simulink model "Modele_LQR_6DOF"  (R2025b)
settings: Solver=VariableStepAuto  StartTime=0.0  StopTime=300  FixedStep=0.033333  RelTol=1e-3
values from neighbouring files (symbols this model uses):
  B = -234.459    [AUV_Params.sldd]    (also in block_compute_K.m = [ [                                          0,             )
  Fx1 = -14.142    [AUV_Params.sldd]
  Fx2 = -14.142    [AUV_Params.sldd]
  Fx3 = 0.0    [AUV_Params.sldd]
  Fx4 = 0.0    [AUV_Params.sldd]
  Fx5 = 0.0    [AUV_Params.sldd]
  Fx6 = 0.0    [AUV_Params.sldd]
  Fx7 = 14.142    [AUV_Params.sldd]
  Fx8 = 14.142    [AUV_Params.sldd]
  Fy1 = 14.142    [AUV_Params.sldd]
  Fy2 = -14.142    [AUV_Params.sldd]
  Fy3 = 0.0    [AUV_Params.sldd]
  Fy4 = 0.0    [AUV_Params.sldd]
  Fy5 = 0.0    [AUV_Params.sldd]
  Fy6 = 0.0    [AUV_Params.sldd]
  Fy7 = 14.142    [AUV_Params.sldd]
  Fy8 = -14.142    [AUV_Params.sldd]
  Fz1 = 0.0    [AUV_Params.sldd]
  Fz2 = 0.0    [AUV_Params.sldd]
  Fz3 = -20.0    [AUV_Params.sldd]
  Fz4 = -20.0    [AUV_Params.sldd]
  Fz5 = -20.0    [AUV_Params.sldd]
  Fz6 = -20.0    [AUV_Params.sldd]
  Fz7 = 0.0    [AUV_Params.sldd]
  Fz8 = 0.0    [AUV_Params.sldd]
  I_x = 0.578    [AUV_Params.sldd]
  I_y = 0.645    [AUV_Params.sldd]
  I_z = 0.9366    [AUV_Params.sldd]
  lx1 = 0.0194    [AUV_Params.sldd]
  lx2 = 0.0194    [AUV_Params.sldd]
  lx3 = -0.0317    [AUV_Params.sldd]
  lx4 = -0.0317    [AUV_Params.sldd]
  lx5 = 0.0317    [AUV_Params.sldd]
  lx6 = 0.0317    [AUV_Params.sldd]
  lx7 = -0.0194    [AUV_Params.sldd]
  lx8 = -0.0194    [AUV_Params.sldd]
  ly1 = 0.0381    [AUV_Params.sldd]
  ly2 = -0.0381    [AUV_Params.sldd]
  ly3 = 0.0049    [AUV_Params.sldd]
  ly4 = -0.0049    [AUV_Params.sldd]
  ly5 = 0.0049    [AUV_Params.sldd]
  ly6 = -0.0049    [AUV_Params.sldd]
  ly7 = 0.0381    [AUV_Params.sldd]
  ly8 = -0.0381    [AUV_Params.sldd]
  lz1 = 0.0575    [AUV_Params.sldd]
  lz2 = 0.0575    [AUV_Params.sldd]
  lz3 = 0.0366    [AUV_Params.sldd]
  lz4 = 0.0366    [AUV_Params.sldd]
  lz5 = 0.0366    [AUV_Params.sldd]
  lz6 = 0.0366    [AUV_Params.sldd]
  lz7 = 0.0575    [AUV_Params.sldd]
  lz8 = 0.0575    [AUV_Params.sldd]
  m = 23.9    [AUV_Params.sldd]
  W = 234.459    [AUV_Params.sldd]
  x_rb = 0.0    [AUV_Params.sldd]
  x_rg = 0.0    [AUV_Params.sldd]
  y_rb = 0.0    [AUV_Params.sldd]
  y_rg = 0.0    [AUV_Params.sldd]
  z_rb = 0.0    [AUV_Params.sldd]
  z_rg = 0.0    [AUV_Params.sldd]
undefined symbols (not defined in the file or in its folder): A_num, Q_envoyer, sigbuilder_block, SIZE_TRAJ, T_TRAJ, TRAJECTOIRE, YAW_MODE
libraries: simulink x12, sharedtransform x1, dspinverses x1, SignalEditorBlockLib x1
(part 2 of 4)

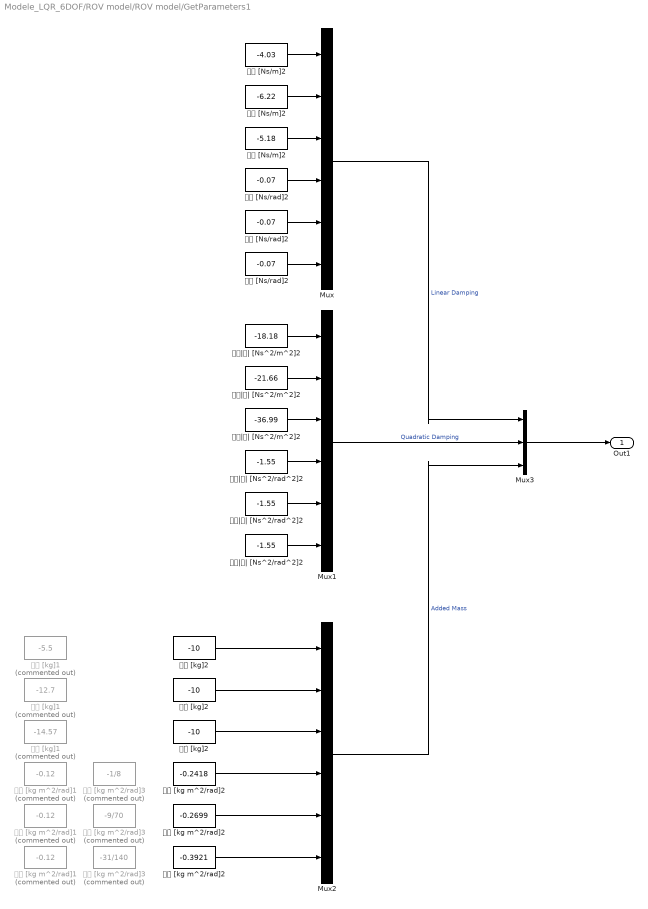
== system Modele_LQR_6DOF/ROV model/ROV model/GetParameters1 ==
  Mux : Mux  Inputs=6
  Mux1 : Mux  Inputs=6
  Mux2 : Mux  Inputs=6
  Mux3 : Mux  Inputs=3
  𝐾𝑝 [Ns/rad]2 : Constant  Value=-0.07
  𝐾𝑝|𝑝| [Ns^2/rad^2]2 : Constant  Value=-1.55
  𝐾𝑝̇ [kg m^2/rad]1 : Constant  Commented=on  Value=-0.12
  𝐾𝑝̇ [kg m^2/rad]2 : Constant  Value=-0.2418
  𝐾𝑝̇ [kg m^2/rad]3 : Constant  Commented=on  Value=-1/8
  𝑀𝑞 [Ns/rad]2 : Constant  Value=-0.07
  𝑀𝑞|𝑞| [Ns^2/rad^2]2 : Constant  Value=-1.55
  𝑀𝑞̇ [kg m^2/rad]1 : Constant  Commented=on  Value=-0.12
  𝑀𝑞̇ [kg m^2/rad]2 : Constant  Value=-0.2699
  𝑀𝑞̇ [kg m^2/rad]3 : Constant  Commented=on  Value=-9/70
  𝑁𝑟 [Ns/rad]2 : Constant  Value=-0.07
  𝑁𝑟|𝑟| [Ns^2/rad^2]2 : Constant  Value=-1.55
  𝑁𝑟̇ [kg m^2/rad]1 : Constant  Commented=on  Value=-0.12
  𝑁𝑟̇ [kg m^2/rad]2 : Constant  Value=-0.3921
  𝑁𝑟̇ [kg m^2/rad]3 : Constant  Commented=on  Value=-31/140
  𝑋𝑢 [Ns/m]2 : Constant  Value=-4.03
  𝑋𝑢|𝑢| [Ns^2/m^2]2 : Constant  Value=-18.18
  𝑋𝑢̇ [kg]1 : Constant  Commented=on  Value=-5.5
  𝑋𝑢̇ [kg]2 : Constant  Value=-10
  𝑌𝑣 [Ns/m]2 : Constant  Value=-6.22
  𝑌𝑣|𝑣| [Ns^2/m^2]2 : Constant  Value=-21.66
  𝑌𝑣̇ [kg]1 : Constant  Commented=on  Value=-12.7
  𝑌𝑣̇ [kg]2 : Constant  Value=-10
  𝑍𝑤 [Ns/m]2 : Constant  Value=-5.18
  𝑍𝑤|𝑤| [Ns^2/m^2]2 : Constant  Value=-36.99
  𝑍𝑤̇ [kg]1 : Constant  Commented=on  Value=-14.57
  𝑍𝑤̇ [kg]2 : Constant  Value=-10
  Out1 : Outport  VectorParamsAs1DForOutWhenUnconnected=off
  wires:
  𝑁𝑟 [Ns/rad]2/1 -> Mux/6
  Mux/1 -> Mux3/1  "Linear Damping"
  𝐾𝑝 [Ns/rad]2/1 -> Mux/4
  𝑀𝑞 [Ns/rad]2/1 -> Mux/5
  𝑍𝑤 [Ns/m]2/1 -> Mux/3
  𝑌𝑣 [Ns/m]2/1 -> Mux/2
  𝑋𝑢 [Ns/m]2/1 -> Mux/1
  𝑌𝑣|𝑣| [Ns^2/m^2]2/1 -> Mux1/2
  𝑍𝑤|𝑤| [Ns^2/m^2]2/1 -> Mux1/3
  𝑋𝑢|𝑢| [Ns^2/m^2]2/1 -> Mux1/1
  Mux1/1 -> Mux3/2  "Quadratic Damping"
  𝑀𝑞|𝑞| [Ns^2/rad^2]2/1 -> Mux1/5
  𝑁𝑟|𝑟| [Ns^2/rad^2]2/1 -> Mux1/6
  𝐾𝑝|𝑝| [Ns^2/rad^2]2/1 -> Mux1/4
  Mux2/1 -> Mux3/3  "Added Mass"
  Mux3/1 -> Out1/1
  𝑋𝑢̇ [kg]2/1 -> Mux2/1
  𝑌𝑣̇ [kg]2/1 -> Mux2/2
  𝑍𝑤̇ [kg]2/1 -> Mux2/3
  𝐾𝑝̇ [kg m^2/rad]2/1 -> Mux2/4
  𝑀𝑞̇ [kg m^2/rad]2/1 -> Mux2/5
  𝑁𝑟̇ [kg m^2/rad]2/1 -> Mux2/6

== matlab function Modele_LQR_6DOF/Controller/Gestionnaire des Vitesses/MATLAB Function1 ==
  data: xstate input; u output; xtarget input
function u = fcn(xstate,xtarget)

precition = 0.01;
% precition = 0.01; % originalt

if(xstate < xtarget - precition)
    u = 1; % original (1)

elseif(xstate > xtarget + precition)
    u = -1; % original (1)
    
else
    u = 0;
end
end

== matlab function Modele_LQR_6DOF/Controller/Gestionnaire des Vitesses/MATLAB Function ==
  data: xstate input; u output; xtarget input
function u = fcn(xstate,xtarget)

precition = 0.01;
% precition = 0.01; % original

if(xstate < xtarget - precition)
    u = 1; % original (1)

elseif(xstate > xtarget + precition)
    u = -1; % original (1)
    
else
    u = 0;
end
end

== matlab function Modele_LQR_6DOF/ROV model/ROV model/Kinetics1 ==
  data: u input size=1; u_dot output; v input size=1; w input size=1; p input size=1; q input size=1; r input size=1; phi input; theta input; psi input; tau input; v_dot output; w_dot output; p_dot output; q_dot output; r_dot output; u_dot_temp input; v_dot_temp input; w_dot_temp input; p_dot_temp input; q_dot_temp input; r_dot_temp input; disturbance input; EstimatedParams input; B parameter; Fx1 input; Fx2 input; Fx3 input; Fx4 input; Fx5 input; Fx6 input; Fx7 input; Fx8 input; Fy1 input; Fy2 input; Fy3 input; Fy4 input; Fy5 input; Fy6 input; Fy7 input; Fy8 input; Fz1 input; Fz2 input; Fz3 input; Fz4 input; Fz5 input; Fz6 input; Fz7 input; Fz8 input; I_x input; I_y input; I_z input; lx1 input; lx2 input; lx3 input; lx4 input; lx5 input; lx6 input; lx7 input; lx8 input; ly1 input; ly2 input; ly3 input; ly4 input; ly5 input; ly6 input; ly7 input; ly8 input; lz1 input; lz2 input; lz3 input; lz4 input; lz5 input; lz6 input; lz7 input; lz8 input; m parameter; W parameter; x_rb parameter; x_rg parameter; y_rb parameter; y_rg parameter; z_rb parameter; z_rg parameter
function [u_dot,v_dot,w_dot,p_dot,q_dot,r_dot] = Kinetics1(u,v,w,p,q,r,phi,theta,psi,tau,u_dot_temp,v_dot_temp,w_dot_temp,p_dot_temp,q_dot_temp,r_dot_temp, disturbance,EstimatedParams, B, Fx1, Fx2, Fx3, Fx4, Fx5, Fx6, Fx7, Fx8, Fy1, Fy2, Fy3, Fy4, Fy5, Fy6, Fy7, Fy8, Fz1, Fz2, Fz3, Fz4, Fz5, Fz6, Fz7, Fz8, I_x, I_y, I_z, lx1, lx2, lx3, lx4, lx5, lx6, lx7, lx8, ly1, ly2, ly3, ly4, ly5, ly6, ly7, ly8, lz1, lz2, lz3, lz4, lz5, lz6, lz7, lz8, m, W, x_rb, x_rg, y_rb, y_rg, z_rb, z_rg)
% LIVRE HMCH PAGE 58
%extract forces from thrusters
f1=tau(1);
f2=tau(2);
f3=tau(3);
f4=tau(4);
f5=tau(5);
f6=tau(6);
f7=tau(7);
f8=tau(8);
x_rb = 0; x_rg = 0; y_rb = 0; y_rg = 0; z_rb = 0; z_rg = 0;
  displaced_water_volume = 0.03; % 0.03
  water_density = 1000.0;
  radius = 0.26;
  m = 23.9;
  g = 9.81;
  W = m * g;
  % B = water_density*displaced_water_volume*g;
  B = W;
%extract estimated parameters
X_u = EstimatedParams(1);
Y_v = EstimatedParams(2);
Z_w = EstimatedParams(3);
K_p = EstimatedParams(4); 
M_q = EstimatedParams(5);
N_r = EstimatedParams(6);
X_uu = EstimatedParams(7);
Y_vv = EstimatedParams(8);
Z_ww = EstimatedParams(9);
K_pp = EstimatedParams(10); 
M_qq = EstimatedParams(11); 
N_rr = EstimatedParams(12);
X_u_dot = EstimatedParams(13);
Y_v_dot = EstimatedParams(14);
Z_w_dot = EstimatedParams(15);
K_p_dot = EstimatedParams(16);
M_q_dot = EstimatedParams(17); 
N_r_dot = EstimatedParams(18); 
%extract forces from disturbance
u_c = disturbance(1);
v_c = disturbance(2);
w_c = disturbance(3);
p_c = disturbance(4);
q_c = disturbance(5);
r_c = disturbance(6);
%Full Equations without disturbance with zg = 0.02
% u_dot = -((0.7071*f1) + (0.7071*f2) - (0.7071*f3) - (0.7071*f4)- (0.230*q_dot_temp) + 2*sin(theta) + u*(X_u + X_uu*abs(u)) - (0.230*p*r) - (11.50*q*w) + (11.50*r*v) - Y_v_dot*r*v + Z_w_dot*q*w)/(X_u_dot - 11.50);
% v_dot = ((0.7071*f1) - (0.7071*f2) + (0.7071*f3) - (0.7071*f4) - (0.230*p_dot_temp) + 2*cos(theta)*sin(phi) - v*(Y_v + Y_vv*abs(v)) + (11.50*q*r) - (11.50*p*w) + (11.50*r*u) - X_u_dot*r*u + Z_w_dot*p*w)/(Y_v_dot - 11.50);
% w_dot = -(f6 - f5 + f7 - f8 - 2*cos(phi)*cos(theta) + w*(Z_w + Z_ww*abs(w)) + q*((23*q)/100 - X_u_dot*u) + p*((23*p)/100 + Y_v_dot*v) - (11.50*p*v) + (11.50*q*u))/(Z_w_dot - 11.50);
% p_dot = -(25*((0.0601*f1) - (0.0601*f2) + (0.0601*f3) - (0.0601*f4) - (109*f5)/500 - (109*f6)/500 + (0.2180*f7) + (0.2180*f8) + (0.230*v_dot_temp) + K_p*p - (2.2560*cos(theta)*sin(phi)) - (0.230*p*w) + (0.230*r*u) - M_q_dot*q*r + N_r_dot*q*r - Y_v_dot*v*w + Z_w_dot*v*w + K_pp*p*abs(p)))/(25*K_p_dot - 4);
% q_dot =-(25*((0.0601*f1) + (0.0601*f2) - (0.0601*f3) - (0.0601*f4)+ (0.120*f5) - (0.120*f6) + (0.120*f7) - (0.120*f8) - (0.230*u_dot_temp) - (2.2560*sin(theta)) + M_q*q - (0.230*q*w) + (0.230*r*v) + K_p_dot*p*r - N_r_dot*p*r + X_u_dot*u*w - Z_w_dot*u*w + M_qq*q*abs(q)))/(25*M_q_dot - 4);
% r_dot = -(25*((0.1888*f2) - (0.1888*f1) + (0.1888*f3) - (0.1888*f4) + N_r*r - K_p_dot*p*q + M_q_dot*p*q - X_u_dot*u*v + Y_v_dot*u*v + N_rr*r*abs(r)))/(25*N_r_dot - 4);

%Full Equations without disturbance with zg = 0.02 + utilisation de la fontion vpa
% u_dot = -(1.0*(0.7071*f1 + 0.7071*f2 - 0.7071*f3 - 0.7071*f4 - 0.23*q_dot_temp + 2.0*sin(theta) + (X_u + X_uu*abs(u - 1.0*u_c))*(u - 1.0*u_c) - 1.0*(11.5*q - 11.5*q_c)*(w - 1.0*w_c) + (11.5*r - 11.5*r_c)*(v - 1.0*v_c) - 1.0*(p - 1.0*p_c)*(0.23*r - 0.23*r_c) + (X_u_dot - 11.5)*(q*w_c - 1.0*r*v_c) - 1.0*Y_v_dot*(r - 1.0*r_c)*(v - 1.0*v_c) + Z_w_dot*(q - 1.0*q_c)*(w - 1.0*w_c)))/(X_u_dot - 11.5);
% v_dot = (0.7071*f1 - 0.7071*f2 + 0.7071*f3 - 0.7071*f4 - 0.23*p_dot_temp - 1.0*(11.5*p - 11.5*p_c)*(w - 1.0*w_c) + (11.5*r - 11.5*r_c)*(u - 1.0*u_c) - 1.0*(Y_v + Y_vv*abs(v - 1.0*v_c))*(v - 1.0*v_c) + 2.0*cos(theta)*sin(phi) + (q - 1.0*q_c)*(0.23*r - 0.23*r_c) + (Y_v_dot - 11.5)*(p*w_c - 1.0*r*u_c) - 1.0*X_u_dot*(r - 1.0*r_c)*(u - 1.0*u_c) + Z_w_dot*(p - 1.0*p_c)*(w - 1.0*w_c))/(Y_v_dot - 11.5);
% w_dot =-(1.0*(f6 - 1.0*f5 + f7 - 1.0*f8 - 1.0*(11.5*p - 11.5*p_c)*(v - 1.0*v_c) + (11.5*q - 11.5*q_c)*(u - 1.0*u_c) - 2.0*cos(phi)*cos(theta) + (Z_w + Z_ww*abs(w - 1.0*w_c))*(w - 1.0*w_c) + (Z_w_dot - 11.5)*(p*v_c - 1.0*q*u_c) + (p - 1.0*p_c)*(0.23*p - 0.23*p_c + Y_v_dot*(v - 1.0*v_c)) - 1.0*(q - 1.0*q_c)*(0.23*q_c - 0.23*q + X_u_dot*(u - 1.0*u_c))))/(Z_w_dot - 11.5);
% p_dot =-(1.0*(0.0601035*f1 - 0.0601035*f2 + 0.0601035*f3 - 0.0601035*f4 - 0.218*f5 - 0.218*f6 + 0.218*f7 + 0.218*f8 + 0.23*v_dot - 2.256*cos(theta)*sin(phi) + (u - 1.0*u_c)*(0.23*r - 0.23*r_c) - 0.23*p*w_c + 0.23*r*u_c - 1.0*(r - 1.0*r_c)*(0.16*q_c - 0.16*q + M_q_dot*(q - 1.0*q_c)) + (q - 1.0*q_c)*(0.16*r_c - 0.16*r + N_r_dot*(r - 1.0*r_c)) + (K_p + K_pp*abs(p - 1.0*p_c))*(p - 1.0*p_c) - 1.0*(w - 1.0*w_c)*(0.23*p - 0.23*p_c + Y_v_dot*(v - 1.0*v_c)) + Z_w_dot*(v - 1.0*v_c)*(w - 1.0*w_c)))/(K_p_dot - 0.16);
% q_dot =-(1.0*(0.0601035*f1 + 0.0601035*f2 - 0.0601035*f3 - 0.0601035*f4 + 0.12*f5 - 0.12*f6 + 0.12*f7 - 0.12*f8 - 0.23*u_dot - 2.256*sin(theta) + (v - 1.0*v_c)*(0.23*r - 0.23*r_c) - 0.23*q*w_c + 0.23*r*v_c + (r - 1.0*r_c)*(0.16*p_c - 0.16*p + K_p_dot*(p - 1.0*p_c)) - 1.0*(p - 1.0*p_c)*(0.16*r_c - 0.16*r + N_r_dot*(r - 1.0*r_c)) + (w - 1.0*w_c)*(0.23*q_c - 0.23*q + X_u_dot*(u - 1.0*u_c)) + (M_q + M_qq*abs(q - 1.0*q_c))*(q - 1.0*q_c) - 1.0*Z_w_dot*(u - 1.0*u_c)*(w - 1.0*w_c)))/(M_q_dot - 0.16);
% r_dot = -(1.0*(0.1887957*f2 - 0.1887957*f1 + 0.1887957*f3 - 0.1887957*f4 - 1.0*(q - 1.0*q_c)*(0.16*p_c - 0.16*p + K_p_dot*(p - 1.0*p_c)) + (p - 1.0*p_c)*(0.16*q_c - 0.16*q + M_q_dot*(q - 1.0*q_c)) + (N_r + N_rr*abs(r - 1.0*r_c))*(r - 1.0*r_c) - 1.0*X_u_dot*(u - 1.0*u_c)*(v - 1.0*v_c) + Y_v_dot*(u - 1.0*u_c)*(v - 1.0*v_c)))/(N_r_dot - 0.16);

% u_dot = -(1.0*((X_u + X_uu*abs(u - 1.0*u_c))*(u - 1.0*u_c) + sin(theta)*(B - 9.81*m) + Fx1*f1 + Fx2*f2 + Fx3*f3 + Fx4*f4 + Fx5*f5 + Fx6*f6 + Fx7*f7 + Fx8*f8 + (q*w_c - 1.0*r*v_c)*(X_u_dot - 1.0*m) + (Z_w_dot*(w - 1.0*w_c) + m*x_rg*(q - 1.0*q_c))*(q - 1.0*q_c) - 1.0*(Y_v_dot*(v - 1.0*v_c) - 1.0*m*x_rg*(r - 1.0*r_c))*(r - 1.0*r_c) - 1.0*(m*y_rg*(q - 1.0*q_c) + m*z_rg*(r - 1.0*r_c))*(p - 1.0*p_c) - 1.0*m*(q - 1.0*q_c)*(w - 1.0*w_c) + m*(r - 1.0*r_c)*(v - 1.0*v_c) - 1.0*m*q_dot_temp*z_rg + m*r_dot_temp*y_rg))/(X_u_dot - 1.0*m);
%  
%  
% v_dot = -(1.0*((Y_v + Y_vv*abs(v - 1.0*v_c))*(v - 1.0*v_c) + Fy1*f1 + Fy2*f2 + Fy3*f3 + Fy4*f4 + Fy5*f5 + Fy6*f6 + Fy7*f7 + Fy8*f8 - 1.0*(p*w_c - 1.0*r*u_c)*(Y_v_dot - 1.0*m) + (X_u_dot*(u - 1.0*u_c) + m*y_rg*(r - 1.0*r_c))*(r - 1.0*r_c) - 1.0*(Z_w_dot*(w - 1.0*w_c) - 1.0*m*y_rg*(p - 1.0*p_c))*(p - 1.0*p_c) - 1.0*(m*x_rg*(p - 1.0*p_c) + m*z_rg*(r - 1.0*r_c))*(q - 1.0*q_c) + m*(p - 1.0*p_c)*(w - 1.0*w_c) - 1.0*m*(r - 1.0*r_c)*(u - 1.0*u_c) + m*p_dot_temp*z_rg - 1.0*m*r_dot_temp*x_rg - 1.0*cos(theta)*sin(phi)*(B - 9.81*m)))/(Y_v_dot - 1.0*m);
%  
%  
% w_dot = -(1.0*(Fz1*f1 + Fz2*f2 + Fz3*f3 + Fz4*f4 + Fz5*f5 + Fz6*f6 + Fz7*f7 + Fz8*f8 + (Z_w + Z_ww*abs(w - 1.0*w_c))*(w - 1.0*w_c) + (p*v_c - 1.0*q*u_c)*(Z_w_dot - 1.0*m) + (Y_v_dot*(v - 1.0*v_c) + m*z_rg*(p - 1.0*p_c))*(p - 1.0*p_c) - 1.0*(X_u_dot*(u - 1.0*u_c) - 1.0*m*z_rg*(q - 1.0*q_c))*(q - 1.0*q_c) - 1.0*(m*x_rg*(p - 1.0*p_c) + m*y_rg*(q - 1.0*q_c))*(r - 1.0*r_c) - 1.0*m*(p - 1.0*p_c)*(v - 1.0*v_c) + m*(q - 1.0*q_c)*(u - 1.0*u_c) - 1.0*m*p_dot_temp*y_rg + m*q_dot_temp*x_rg - 1.0*cos(phi)*cos(theta)*(B - 9.81*m)))/(Z_w_dot - 1.0*m);
%  
%  
% p_dot = -(1.0*((Y_v_dot*(v - 1.0*v_c) + m*z_rg*(p - 1.0*p_c))*(w - 1.0*w_c) + f1*(Fy1*lz1 - 1.0*Fz1*ly1) + f2*(Fy2*lz2 - 1.0*Fz2*ly2) + f3*(Fy3*lz3 - 1.0*Fz3*ly3) + f4*(Fy4*lz4 - 1.0*Fz4*ly4) + f5*(Fy5*lz5 - 1.0*Fz5*ly5) + f6*(Fy6*lz6 - 1.0*Fz6*ly6) + f7*(Fy7*lz7 - 1.0*Fz7*ly7) + f8*(Fy8*lz8 - 1.0*Fz8*ly8) - 1.0*(Z_w_dot*(w - 1.0*w_c) - 1.0*m*y_rg*(p - 1.0*p_c))*(v - 1.0*v_c) - 1.0*(K_p + K_pp*abs(p - 1.0*p_c))*(p - 1.0*p_c) - 1.0*(m*y_rg*(q - 1.0*q_c) + m*z_rg*(r - 1.0*r_c))*(u - 1.0*u_c) - 1.0*(I_y*(q - 1.0*q_c) - 1.0*M_q_dot*(q - 1.0*q_c))*(r - 1.0*r_c) + (I_z*(r - 1.0*r_c) - 1.0*N_r_dot*(r - 1.0*r_c))*(q - 1.0*q_c) + cos(phi)*cos(theta)*(B*y_rb - 9.81*m*y_rg) - 1.0*cos(theta)*sin(phi)*(B*z_rb - 9.81*m*z_rg) + m*y_rg*(w_dot + p*v_c - 1.0*q*u_c) - 1.0*m*z_rg*(v_dot - 1.0*p*w_c + r*u_c)))/(I_x - 1.0*K_p_dot);
%  
%  
% q_dot = (sin(theta)*(B*z_rb - 9.81*m*z_rg) - 1.0*(Z_w_dot*(w - 1.0*w_c) + m*x_rg*(q - 1.0*q_c))*(u - 1.0*u_c) + f1*(Fx1*lz1 - 1.0*Fz1*lx1) + f2*(Fx2*lz2 - 1.0*Fz2*lx2) + f3*(Fx3*lz3 - 1.0*Fz3*lx3) + f4*(Fx4*lz4 - 1.0*Fz4*lx4) + f5*(Fx5*lz5 - 1.0*Fz5*lx5) + f6*(Fx6*lz6 - 1.0*Fz6*lx6) + f7*(Fx7*lz7 - 1.0*Fz7*lx7) + f8*(Fx8*lz8 - 1.0*Fz8*lx8) + (X_u_dot*(u - 1.0*u_c) - 1.0*m*z_rg*(q - 1.0*q_c))*(w - 1.0*w_c) + (M_q + M_qq*abs(q - 1.0*q_c))*(q - 1.0*q_c) - 1.0*(I_x*(p - 1.0*p_c) - 1.0*K_p_dot*(p - 1.0*p_c))*(r - 1.0*r_c) + (m*x_rg*(p - 1.0*p_c) + m*z_rg*(r - 1.0*r_c))*(v - 1.0*v_c) + (I_z*(r - 1.0*r_c) - 1.0*N_r_dot*(r - 1.0*r_c))*(p - 1.0*p_c) + cos(phi)*cos(theta)*(B*x_rb - 9.81*m*x_rg) + m*x_rg*(w_dot + p*v_c - 1.0*q*u_c) - 1.0*m*z_rg*(u_dot + q*w_c - 1.0*r*v_c))/(I_y - 1.0*M_q_dot);
%  
%  
% r_dot = -(1.0*(sin(theta)*(B*y_rb - 9.81*m*y_rg) + (X_u_dot*(u - 1.0*u_c) + m*y_rg*(r - 1.0*r_c))*(v - 1.0*v_c) + f1*(Fx1*ly1 - 1.0*Fy1*lx1) + f2*(Fx2*ly2 - 1.0*Fy2*lx2) + f3*(Fx3*ly3 - 1.0*Fy3*lx3) + f4*(Fx4*ly4 - 1.0*Fy4*lx4) + f5*(Fx5*ly5 - 1.0*Fy5*lx5) + f6*(Fx6*ly6 - 1.0*Fy6*lx6) + f7*(Fx7*ly7 - 1.0*Fy7*lx7) + f8*(Fx8*ly8 - 1.0*Fy8*lx8) - 1.0*(Y_v_dot*(v - 1.0*v_c) - 1.0*m*x_rg*(r - 1.0*r_c))*(u - 1.0*u_c) - 1.0*(N_r + N_rr*abs(r - 1.0*r_c))*(r - 1.0*r_c) - 1.0*(I_x*(p - 1.0*p_c) - 1.0*K_p_dot*(p - 1.0*p_c))*(q - 1.0*q_c) + (I_y*(q - 1.0*q_c) - 1.0*M_q_dot*(q - 1.0*q_c))*(p - 1.0*p_c) - 1.0*(m*x_rg*(p - 1.0*p_c) + m*y_rg*(q - 1.0*q_c))*(w - 1.0*w_c) + cos(theta)*sin(phi)*(B*x_rb - 9.81*m*x_rg) + m*x_rg*(v_dot - 1.0*p*w_c + r*u_c) - 1.0*m*y_rg*(u_dot + q*w_c - 1.0*r*v_c)))/(I_z - 1.0*N_r_dot);
%-------------------------------------------------------------------------------------------------------------------------------------------------------------------------------------------------------------------------------------------------------------------------------------------------------------------------------------------------------------------------------------------------------------------------------------------------------------------------------------------------------------------------------------------------------------% 
u_dot = -(1.0*((X_u + X_uu*abs(u - 1.0*u_c))*(u - 1.0*u_c) + Fx1*f1 + Fx2*f2 + Fx3*f3 + Fx4*f4 + Fx5*f5 + Fx6*f6 + Fx7*f7 + Fx8*f8 + (q*w_c - 1.0*r*v_c)*(X_u_dot - 1.0*m) + (Z_w_dot*(w - 1.0*w_c) + m*x_rg*(q - 1.0*q_c))*(q - 1.0*q_c) - 1.0*(Y_v_dot*(v - 1.0*v_c) - 1.0*m*x_rg*(r - 1.0*r_c))*(r - 1.0*r_c) + sin(theta)*(B - 1.0*W) - 1.0*(m*y_rg*(q - 1.0*q_c) + m*z_rg*(r - 1.0*r_c))*(p - 1.0*p_c) - 1.0*m*(q - 1.0*q_c)*(w - 1.0*w_c) + m*(r - 1.0*r_c)*(v - 1.0*v_c) - 1.0*m*q_dot_temp*z_rg + m*r_dot_temp*y_rg))/(X_u_dot - 1.0*m);


v_dot = -(1.0*((Y_v + Y_vv*abs(v - 1.0*v_c))*(v - 1.0*v_c) + Fy1*f1 + Fy2*f2 + Fy3*f3 + Fy4*f4 + Fy5*f5 + Fy6*f6 + Fy7*f7 + Fy8*f8 - 1.0*(p*w_c - 1.0*r*u_c)*(Y_v_dot - 1.0*m) + (X_u_dot*(u - 1.0*u_c) + m*y_rg*(r - 1.0*r_c))*(r - 1.0*r_c) - 1.0*(Z_w_dot*(w - 1.0*w_c) - 1.0*m*y_rg*(p - 1.0*p_c))*(p - 1.0*p_c) - 1.0*(m*x_rg*(p - 1.0*p_c) + m*z_rg*(r - 1.0*r_c))*(q - 1.0*q_c) + m*(p - 1.0*p_c)*(w - 1.0*w_c) - 1.0*m*(r - 1.0*r_c)*(u - 1.0*u_c) - 1.0*cos(theta)*sin(phi)*(B - 1.0*W) + m*p_dot_temp*z_rg - 1.0*m*r_dot_temp*x_rg))/(Y_v_dot - 1.0*m);


w_dot = -(1.0*(Fz1*f1 + Fz2*f2 + Fz3*f3 + Fz4*f4 + Fz5*f5 + Fz6*f6 + Fz7*f7 + Fz8*f8 + (Z_w + Z_ww*abs(w - 1.0*w_c))*(w - 1.0*w_c) + (p*v_c - 1.0*q*u_c)*(Z_w_dot - 1.0*m) + (Y_v_dot*(v - 1.0*v_c) + m*z_rg*(p - 1.0*p_c))*(p - 1.0*p_c) - 1.0*(X_u_dot*(u - 1.0*u_c) - 1.0*m*z_rg*(q - 1.0*q_c))*(q - 1.0*q_c) - 1.0*(m*x_rg*(p - 1.0*p_c) + m*y_rg*(q - 1.0*q_c))*(r - 1.0*r_c) - 1.0*m*(p - 1.0*p_c)*(v - 1.0*v_c) + m*(q - 1.0*q_c)*(u - 1.0*u_c) - 1.0*cos(phi)*cos(theta)*(B - 1.0*W) - 1.0*m*p_dot_temp*y_rg + m*q_dot_temp*x_rg))/(Z_w_dot - 1.0*m);


p_dot = -(1.0*((Y_v_dot*(v - 1.0*v_c) + m*z_rg*(p - 1.0*p_c))*(w - 1.0*w_c) - 1.0*cos(theta)*(W*y_rg*cos(phi) - 1.0*W*z_rg*sin(phi) - 1.0*B*y_rb*cos(phi) + B*z_rb*sin(phi)) + f1*(Fy1*lz1 - 1.0*Fz1*ly1) + f2*(Fy2*lz2 - 1.0*Fz2*ly2) + f3*(Fy3*lz3 - 1.0*Fz3*ly3) + f4*(Fy4*lz4 - 1.0*Fz4*ly4) + f5*(Fy5*lz5 - 1.0*Fz5*ly5) + f6*(Fy6*lz6 - 1.0*Fz6*ly6) + f7*(Fy7*lz7 - 1.0*Fz7*ly7) + f8*(Fy8*lz8 - 1.0*Fz8*ly8) - 1.0*(Z_w_dot*(w - 1.0*w_c) - 1.0*m*y_rg*(p - 1.0*p_c))*(v - 1.0*v_c) - 1.0*(K_p + K_pp*abs(p - 1.0*p_c))*(p - 1.0*p_c) - 1.0*(m*y_rg*(q - 1.0*q_c) + m*z_rg*(r - 1.0*r_c))*(u - 1.0*u_c) - 1.0*(I_y*(q - 1.0*q_c) - 1.0*M_q_dot*(q - 1.0*q_c))*(r - 1.0*r_c) + (I_z*(r - 1.0*r_c) - 1.0*N_r_dot*(r - 1.0*r_c))*(q - 1.0*q_c) + m*y_rg*(w_dot + p*v_c - 1.0*q*u_c) - 1.0*m*z_rg*(v_dot - 1.0*p*w_c + r*u_c)))/(I_x - 1.0*K_p_dot);


q_dot = (f1*(Fx1*lz1 - 1.0*Fz1*lx1) - 1.0*(Z_w_dot*(w - 1.0*w_c) + m*x_rg*(q - 1.0*q_c))*(u - 1.0*u_c) + f2*(Fx2*lz2 - 1.0*Fz2*lx2) + f3*(Fx3*lz3 - 1.0*Fz3*lx3) + f4*(Fx4*lz4 - 1.0*Fz4*lx4) + f5*(Fx5*lz5 - 1.0*Fz5*lx5) + f6*(Fx6*lz6 - 1.0*Fz6*lx6) + f7*(Fx7*lz7 - 1.0*Fz7*lx7) + f8*(Fx8*lz8 - 1.0*Fz8*lx8) + (X_u_dot*(u - 1.0*u_c) - 1.0*m*z_rg*(q - 1.0*q_c))*(w - 1.0*w_c) + (M_q + M_qq*abs(q - 1.0*q_c))*(q - 1.0*q_c) - 1.0*(I_x*(p - 1.0*p_c) - 1.0*K_p_dot*(p - 1.0*p_c))*(r - 1.0*r_c) + (m*x_rg*(p - 1.0*p_c) + m*z_rg*(r - 1.0*r_c))*(v - 1.0*v_c) + (I_z*(r - 1.0*r_c) - 1.0*N_r_dot*(r - 1.0*r_c))*(p - 1.0*p_c) + B*z_rb*sin(theta) - 1.0*W*z_rg*sin(theta) + m*x_rg*(w_dot + p*v_c - 1.0*q*u_c) - 1.0*m*z_rg*(u_dot + q*w_c - 1.0*r*v_c) + B*x_rb*cos(phi)*cos(theta) - 1.0*W*x_rg*cos(phi)*cos(theta))/(I_y - 1.0*M_q_dot);


r_dot = -(1.0*((X_u_dot*(u - 1.0*u_c) + m*y_rg*(r - 1.0*r_c))*(v - 1.0*v_c) + f1*(Fx1*ly1 - 1.0*Fy1*lx1) + f2*(Fx2*ly2 - 1.0*Fy2*lx2) + f3*(Fx3*ly3 - 1.0*Fy3*lx3) + f4*(Fx4*ly4 - 1.0*Fy4*lx4) + f5*(Fx5*ly5 - 1.0*Fy5*lx5) + f6*(Fx6*ly6 - 1.0*Fy6*lx6) + f7*(Fx7*ly7 - 1.0*Fy7*lx7) + f8*(Fx8*ly8 - 1.0*Fy8*lx8) - 1.0*(Y_v_dot*(v - 1.0*v_c) - 1.0*m*x_rg*(r - 1.0*r_c))*(u - 1.0*u_c) - 1.0*(N_r + N_rr*abs(r - 1.0*r_c))*(r - 1.0*r_c) - 1.0*(I_x*(p - 1.0*p_c) - 1.0*K_p_dot*(p - 1.0*p_c))*(q - 1.0*q_c) + (I_y*(q - 1.0*q_c) - 1.0*M_q_dot*(q - 1.0*q_c))*(p - 1.0*p_c) - 1.0*(m*x_rg*(p - 1.0*p_c) + m*y_rg*(q - 1.0*q_c))*(w - 1.0*w_c) + B*y_rb*sin(theta) - 1.0*W*y_rg*sin(theta) + m*x_rg*(v_dot - 1.0*p*w_c + r*u_c) - 1.0*m*y_rg*(u_dot + q*w_c - 1.0*r*v_c) + B*x_rb*cos(theta)*sin(phi) - 1.0*W*x_rg*cos(theta)*sin(phi)))/(I_z - 1.0*N_r_dot);
%-------------------------------------------------------------------------------------------------------------------------------------------------------------------------------------------------------------------------------------------------------------------------------------------------------------------------------------------------------------------------------------------------------------------------------------------------------------------------------------------------------------------------------------------------------------% 

end
